simulink model "SWC_DKC_type"  (R2021b)
settings: Solver=FixedStepDiscrete  StartTime=0.0  StopTime=10.0  FixedStep=0.01  RelTol=1e-3
settings Model: DataDictionary=APPTypes.sldd  Creator=FVT24007  LastModifiedBy=FVT22063
settings DataIOCC: SaveFormat=StructureWithTime
settings OptimizationCC: DefaultParameterBehavior=Inlined  EnhancedBackFolding=on  PassReuseOutputArgsAs=Individual arguments  ZeroExternalMemoryAtStartup=off  ZeroInternalMemoryAtStartup=off  OptimizeBlockOrder=speed  DifferentSizesBufferReuse=on  OptimizationCustomize=off  EfficientTunableParamExpr=on
settings DebuggingCC: ParameterTunabilityLossMsg=error
settings HardwareCC: ProdBitPerPointer=32  ProdBitPerSizeT=32  ProdBitPerPtrDiffT=32  ProdLargestAtomicInteger=Long  ProdLargestAtomicFloat=Double  ProdWordSize=32  ProdLongLongMode=on  ProdHWDeviceType=ARM Compatible->ARM Cortex-M
settings ModelReferenceCC: ModelReferenceNumInstancesAllowed=Single
settings SFSimCC: MATLABDynamicMemAlloc=off
settings RTWCC: Description=AUTOSAR  SystemTargetFile=autosar.tlc  GenCodeOnly=on  TemplateMakefile=ert_default_tmf  PortableWordSizes=on
settings CodeAppCC: ForceParamTrailComments=on  IgnoreCustomStorageClasses=off  OperatorAnnotations=on  SimulinkDataObjDesc=on  SFDataObjDesc=on  InsertBlockDesc=on
settings STFCustomTargetCC: TargetLangStandard=C99 (ISO)  UtilityFuncGeneration=Shared location  MultiwordLength=256  ParMdlRefBuildCompliant=on  CompOptLevelCompliant=on  IncludeMdlTerminateFcn=off  CombineOutputUpdateFcns=on  SuppressErrorStatus=on  ERTCustomFileBanners=on  SupportNonFinite=off  SupportComplex=off  SupportContinuousTime=off  SupportNonInlinedSFcns=off  RemoveResetFunc=on  MATLABClassNameForMDSCustomization=Simulink.SoftwareTarget.ERTCustomization  AutosarCompliant=on  GRTInterface=off  UseToolchainInfoCompliant=on  GenerateSharedConstants=off  LookupTableObjectStructAxisOrder=2,1,3,4,...  LUTObjectStructOrderEvenSpacing=Size,Table,Breakpoints  SystemTargetFile=autosar.tlc
settings ERTTargetCC: TargetLangStandard=C99 (ISO)  UtilityFuncGeneration=Shared location  ConcurrentExecutionCompliant=off  IncludeMdlTerminateFcn=off  SuppressErrorStatus=on  SupportNonFinite=off  SupportComplex=off  ModelStepFunctionPrototypeControlCompliant=off  CPPClassGenCompliant=off  AutosarCompliant=on  GenerateSharedConstants=off  LookupTableObjectStructAxisOrder=2,1,3,4,...  LUTObjectStructOrderEvenSpacing=Size,Table,Breakpoints  GenerateASAP2=on  InlinedParameterPlacement=NonHierarchical  ERTCustomFileTemplate=example_file_process.tlc  ConvertIfToSwitch=off  SuppressUnreachableDefaultCases=off  BooleanTrueId=true_MatlabRTW  BooleanFalseId=false_MatlabRTW

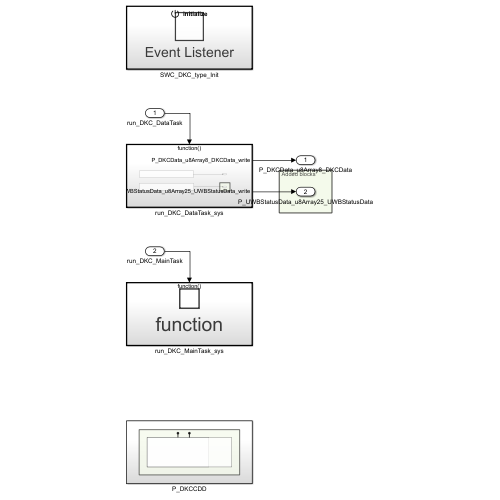
[thumbnail: Simulink's stored preview of the top-level diagram]
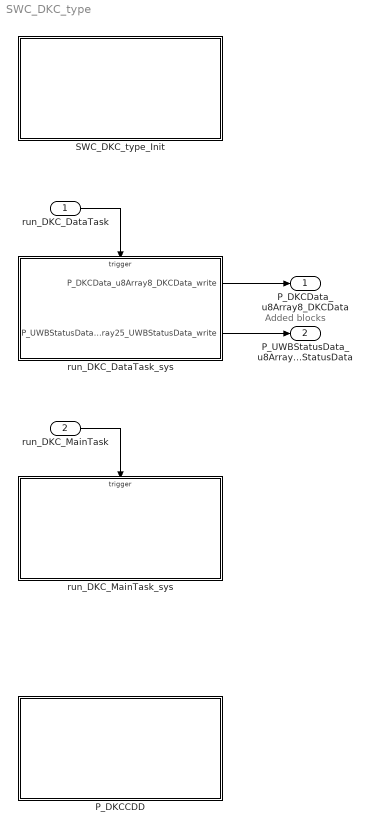
== system SWC_DKC_type ==
  note: Added blocks
  run_DKC_DataTask : Inport  SampleTime=0.1  OutputFunctionCall=on
  run_DKC_MainTask : Inport  Port=2  SampleTime=0.01  OutputFunctionCall=on
  P_DKCCDD : Subsystem
  SWC_DKC_type_Init : Subsystem
  run_DKC_DataTask_sys : Subsystem
  run_DKC_MainTask_sys : Subsystem
  P_DKCData_u8Array8_DKCData : Outport  OutDataTypeStr=uint8  PortDimensions=8
  P_UWBStatusData_u8Array25_UWBStatusData : Outport  Port=2  OutDataTypeStr=uint8  PortDimensions=25
  wires:
  run_DKC_DataTask_sys/1(P_DKCData_u8Array8_DKCData_write) -> P_DKCData_u8Array8_DKCData/1
  run_DKC_DataTask/1 -> run_DKC_DataTask_sys/Trigger
  run_DKC_MainTask/1 -> run_DKC_MainTask_sys/Trigger
  run_DKC_DataTask_sys/2(P_UWBStatusData_u8Array25_UWBStatusData_write) -> P_UWBStatusData_u8Array25_UWBStatusData/1

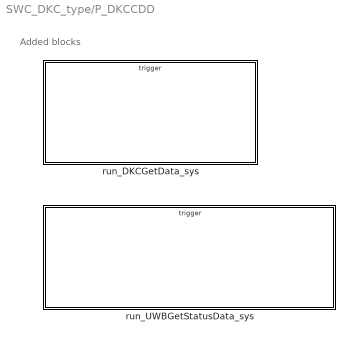
== system SWC_DKC_type/P_DKCCDD ==
  note: Added blocks
  run_DKCGetData_sys : Subsystem
  run_UWBGetStatusData_sys : Subsystem

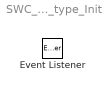
== system SWC_DKC_type/SWC_DKC_type_Init ==
  Event Listener : EventListener  EventName=reset

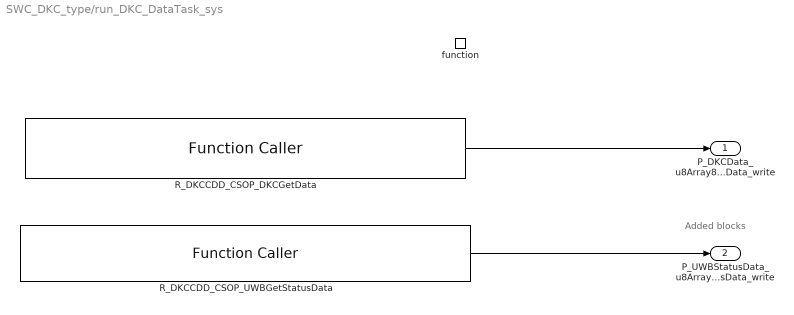
== system SWC_DKC_type/run_DKC_DataTask_sys ==
  note: Added blocks
  function : TriggerPort  TriggerType=function-call  VariantControl=(inherit)  SampleTimeType=periodic  SampleTime=-1
  R_DKCCDD_CSOP_DKCGetData : FunctionCaller  FunctionPrototype=u8Array8_DKCData = R_DKCCDD_CSOP_DKCGetData()  OutputArgumentSpecifications=uint8([1;1;1;1;1;1;1;1])
  R_DKCCDD_CSOP_UWBGetStatusData : FunctionCaller  FunctionPrototype=u8Array25_UWBStatusData = R_DKCCDD_CSOP_UWBGetStatusData()  OutputArgumentSpecifications=uint8([1;1;1;1;1;1;1;1;1;1;1;1;1;1;1;1;1;1;1;1;1;1;1;1;1])
  P_DKCData_u8Array8_DKCData_write : Outport
  P_UWBStatusData_u8Array25_UWBStatusData_write : Outport  Port=2
  wires:
  R_DKCCDD_CSOP_DKCGetData/1 -> P_DKCData_u8Array8_DKCData_write/1
  R_DKCCDD_CSOP_UWBGetStatusData/1 -> P_UWBStatusData_u8Array25_UWBStatusData_write/1

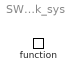
== system SWC_DKC_type/run_DKC_MainTask_sys ==
  function : TriggerPort  TriggerType=function-call  VariantControl=(inherit)  SampleTimeType=periodic  SampleTime=-1

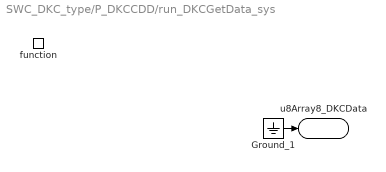
== system SWC_DKC_type/P_DKCCDD/run_DKCGetData_sys ==
  function : TriggerPort  TriggerType=function-call  IsSimulinkFunction=on  FunctionName=run_DKCGetData  VariantControl=(inherit)
  Ground_1 : Ground
  u8Array8_DKCData : ArgOut  OutDataTypeStr=uint8  PortDimensions=8  ArgumentName=u8Array8_DKCData
  wires:
  Ground_1/1 -> u8Array8_DKCData/1

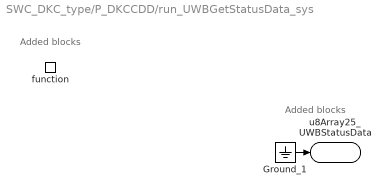
== system SWC_DKC_type/P_DKCCDD/run_UWBGetStatusData_sys ==
  note: Added blocks
  note: Added blocks
  function : TriggerPort  TriggerType=function-call  IsSimulinkFunction=on  FunctionName=run_UWBGetStatusData  VariantControl=(inherit)
  Ground_1 : Ground
  u8Array25_UWBStatusData : ArgOut  OutDataTypeStr=uint8  PortDimensions=25  ArgumentName=u8Array25_UWBStatusData
  wires:
  Ground_1/1 -> u8Array25_UWBStatusData/1
